simulink model "blocks"  (R2017b)
settings: Solver=VariableStepAuto  StartTime=0.0  StopTime=10.0  RelTol=1e-3
settings Model: Creator=riccardoferrar  LastModifiedBy=riccardoferrar

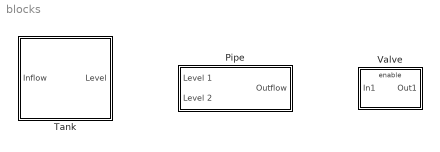
== system blocks ==
  Pipe : Subsystem  mask(Connection Pipe){S_p=1, c_o=1}
      mask prompts: S_p "Pipe cross-section [m^2]"; c_o "Outflow coefficient"
      mask help:
      | Connection pipe between two tanks.
      | The pipe cross-section and the outflow coefficient are mask block parameters.
      mask Help:
      | Enter the pipe cross-section [S_p] and the outflow coefficient [c_o] in the block dialog parameter fields.
      | 
      | The block generates the pipe's flow-rate. The input signals are the level of fluid into both the tanks, connected by the pipe. If the level in the first tank is bigger than the level in the second one, the fluid flow from the first to the second tank, else in the opposite way.
      mask Display: image(imread('pipe.jpg'));
  Tank : Subsystem  mask(Tank system){S=1, x_0=0.5, max_level=1, min_level=0}
      mask prompts: S "Tank cross-section [m^2]"; x_0 "Initial fluid level [m"; max_level "Maximum fluid level [m]"; min_level "Minimum fluid level [m]"
      mask help:
      | Model of  a simple tank system. The input is a fluid flow-rate (may be positive or negative), the output is the fluid level in the tank.
      |
      | The tank cross-section, the initial, minimum and maximum fluid level are mask block parameters.
      mask Help:
      | Enter the tank cross-section, the initial, minimum, maximum fluid level in the block dialog parameter fields.
      | 
      | The block models a simple tank system. The input is the fluid flow-rate (positive or negative) that feeds the system; the output is the fluid level in the tank.
      mask Display: image(imread('tank.jpg'));
  Valve : Subsystem  TreatAsAtomicUnit=on  mask(Valve subsystem){}
      mask help: Model of a valve. When the control signal is greather then 0, the output is equal to the input. Otherwise, the output is 0.
      mask Display: image(imread('valve.jpg'))

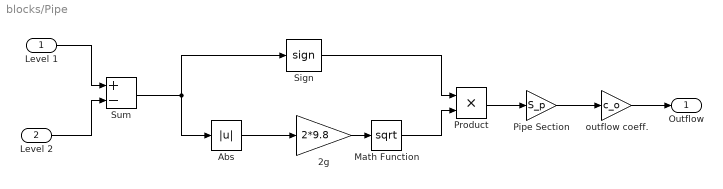
== system blocks/Pipe ==
  Level 1 : Inport
  Level 2 : Inport  Port=2
  2g : Gain  Gain=2*9.8  SaturateOnIntegerOverflow=on  OutDataTypeStr=Inherit: Same as input  ParamDataTypeStr=Inherit: Same as input
  Abs : Abs  SaturateOnIntegerOverflow=on
  Math Function : Math  Operator=sqrt  SaturateOnIntegerOverflow=on
  Pipe Section : Gain  Gain=S_p  SaturateOnIntegerOverflow=on  OutDataTypeStr=Inherit: Same as input  ParamDataTypeStr=Inherit: Same as input
  Product : Product  SaturateOnIntegerOverflow=on  InputSameDT=on  OutDataTypeStr=Inherit: Same as first input
  Sign : Signum
  Sum : Sum  Inputs=+-  SaturateOnIntegerOverflow=on  InputSameDT=on  OutDataTypeStr=Inherit: Same as first input
  outflow coeff. : Gain  Gain=c_o  SaturateOnIntegerOverflow=on  OutDataTypeStr=Inherit: Same as input  ParamDataTypeStr=Inherit: Same as input
  Outflow : Outport
  wires:
  Level 1/1 -> Sum/1
  Level 2/1 -> Sum/2
  Sum/1 -> Sign/1, Abs/1
  Abs/1 -> 2g/1
  2g/1 -> Math Function/1
  Math Function/1 -> Product/2
  Sign/1 -> Product/1
  Product/1 -> Pipe Section/1
  Pipe Section/1 -> outflow coeff./1
  outflow coeff./1 -> Outflow/1

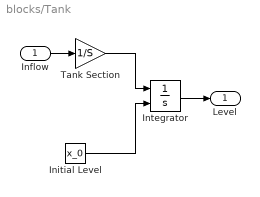
== system blocks/Tank ==
  Inflow : Inport
  Initial Level : Constant  Value=x_0
  Integrator : Integrator  InitialConditionSource=external  LimitOutput=on  UpperSaturationLimit=max_level  LowerSaturationLimit=min_level
  Tank Section : Gain  Gain=1/S  SaturateOnIntegerOverflow=on  OutDataTypeStr=Inherit: Same as input  ParamDataTypeStr=Inherit: Same as input
  Level : Outport  InitialOutput=0
  wires:
  Inflow/1 -> Tank Section/1
  Tank Section/1 -> Integrator/1
  Initial Level/1 -> Integrator/2
  Integrator/1 -> Level/1

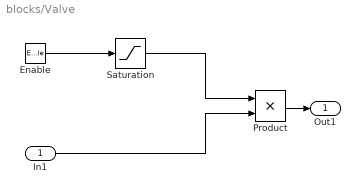
== system blocks/Valve ==
  In1 : Inport
  Enable : EnablePort  StatesWhenEnabling=reset  ShowOutputPort=on
  Product : Product  SaturateOnIntegerOverflow=on  InputSameDT=on  OutDataTypeStr=Inherit: Same as first input
  Saturation : Saturate  UpperLimit=1.0  LowerLimit=0.0
  Out1 : Outport
  wires:
  Enable/1 -> Saturation/1
  Saturation/1 -> Product/1
  In1/1 -> Product/2
  Product/1 -> Out1/1
